simulink model "ME419_Ex1_7"  (R2023b)
settings: Solver=VariableStepAuto  StartTime=0.0  StopTime=80  RelTol=1e-6
settings Model: Creator=aliawolken  LastModifiedBy=aliawolken

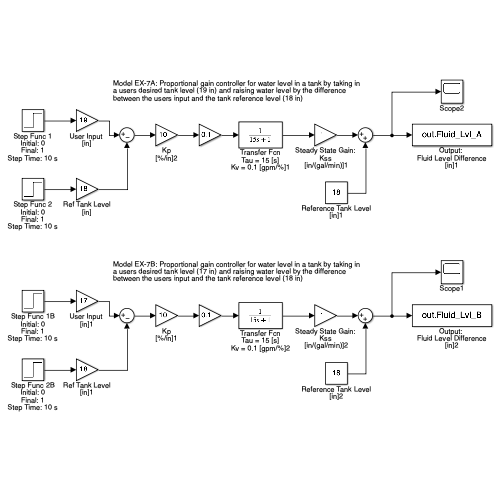
[thumbnail: Simulink's stored preview of the top-level diagram]
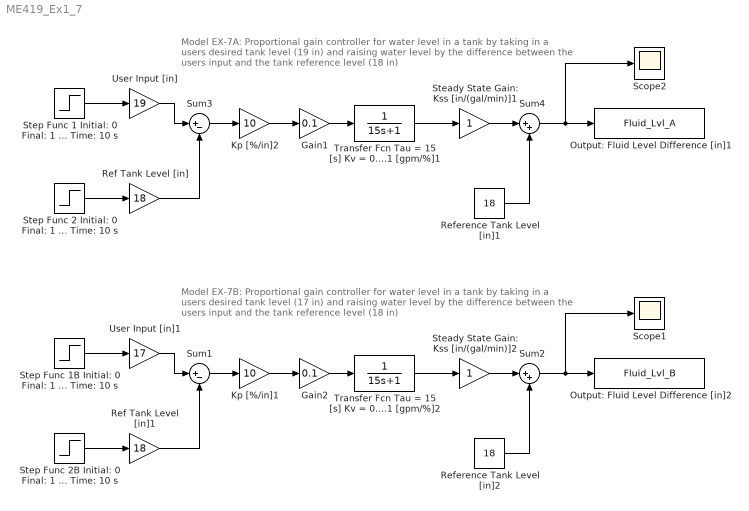
== system ME419_Ex1_7 ==
  note: Model EX-7A: Proportional gain controller for water level in a tank by taking in a users desired tank level (19 in) and raising water level by the difference between the users input and the tank reference level (18 in)
  note: Model EX-7B: Proportional gain controller for water level in a tank by taking in a users desired tank level (17 in) and raising water level by the difference between the users input and the tank reference level (18 in)
  Gain1 : Gain  Gain=0.1
  Gain2 : Gain  Gain=0.1
  Kp [%/in]1 : Gain  Gain=10
  Kp [%/in]2 : Gain  Gain=10
  Output: Fluid Level Difference [in]1 : ToWorkspace  VariableName=Fluid_Lvl_A  SampleTime=-1
  Output: Fluid Level Difference [in]2 : ToWorkspace  VariableName=Fluid_Lvl_B  SampleTime=-1
  Ref Tank Level [in] : Gain  Gain=18
  Ref Tank Level [in]1 : Gain  Gain=18
  Reference Tank Level [in]1 : Constant  Value=18
  Reference Tank Level [in]2 : Constant  Value=18
  Scope1 : Scope
  Scope2 : Scope
  Steady State Gain: Kss [in/(gal/min)]1 : Gain
  Steady State Gain: Kss [in/(gal/min)]2 : Gain
  Step Func 1 Initial: 0 Final: 1 Step Time: 10 s : Step  Time=10  SampleTime=0
  Step Func 1B Initial: 0 Final: 1 Step Time: 10 s : Step  Time=10  SampleTime=0
  "Step Func 2 Initial: 0 Final: 1 Step Time: 10 s " : Step  Time=10  SampleTime=0
  "Step Func 2B Initial: 0 Final: 1 Step Time: 10 s " : Step  Time=10  SampleTime=0
  Sum1 : Sum  Inputs=|+-
  Sum2 : Sum  Inputs=|++
  Sum3 : Sum  Inputs=|+-
  Sum4 : Sum  Inputs=|++
  Transfer Fcn Tau = 15 [s] Kv = 0.1 [gpm/%]1 : TransferFcn  Denominator=[15 1]
  Transfer Fcn Tau = 15 [s] Kv = 0.1 [gpm/%]2 : TransferFcn  Denominator=[15 1]
  User Input [in] : Gain  Gain=19
  User Input [in]1 : Gain  Gain=17
  wires:
  Gain1/1 -> Transfer Fcn Tau = 15 [s] Kv = 0.1 [gpm/%]1/1
  Kp [%/in]2/1 -> Gain1/1
  Transfer Fcn Tau = 15 [s] Kv = 0.1 [gpm/%]1/1 -> Steady State Gain: Kss [in/(gal/min)]1/1
  Sum3/1 -> Kp [%/in]2/1
  Steady State Gain: Kss [in/(gal/min)]1/1 -> Sum4/1
  Sum4/1 -> Scope2/1, Output: Fluid Level Difference [in]1/1
  Reference Tank Level [in]1/1 -> Sum4/2
  User Input [in]/1 -> Sum3/1
  Step Func 1 Initial: 0 Final: 1 Step Time: 10 s/1 -> User Input [in]/1
  Ref Tank Level [in]/1 -> Sum3/2
  "Step Func 2 Initial: 0 Final: 1 Step Time: 10 s "/1 -> Ref Tank Level [in]/1
  Gain2/1 -> Transfer Fcn Tau = 15 [s] Kv = 0.1 [gpm/%]2/1
  Kp [%/in]1/1 -> Gain2/1
  Sum1/1 -> Kp [%/in]1/1
  Steady State Gain: Kss [in/(gal/min)]2/1 -> Sum2/1
  Transfer Fcn Tau = 15 [s] Kv = 0.1 [gpm/%]2/1 -> Steady State Gain: Kss [in/(gal/min)]2/1
  Sum2/1 -> Scope1/1, Output: Fluid Level Difference [in]2/1
  Ref Tank Level [in]1/1 -> Sum1/2
  Reference Tank Level [in]2/1 -> Sum2/2
  User Input [in]1/1 -> Sum1/1
  Step Func 1B Initial: 0 Final: 1 Step Time: 10 s/1 -> User Input [in]1/1
  "Step Func 2B Initial: 0 Final: 1 Step Time: 10 s "/1 -> Ref Tank Level [in]1/1
